simulink model "Project2"  (Simulink 8.0)
settings: Solver=ode23s  StartTime=0.0  StopTime=600  RelTol=1e-4
values from neighbouring files (symbols this model uses):
  a_1 = X(1)    [Init_Project1.m]
  a_2 = X(2)    [Init_Project1.m]
  a_3 = X(3)    [Init_Project1.m]
  A_max_wg = 0.035^2/4*pi    (= 0.000962112750162)    [Init_Project2.m]
  AFS = EngineMap.airfuel.AFs    [Init_Project1.m]
  alpha_REF_manual = 0    [Init_Project2.m]
  alphaEND = alphaINI    (= 0.1)    [Init_Project2.m]
  alphaINI = 0.1    [Init_Project2.m]
  alphaST = 0    [Init_Project2.m]
  BSR_max = turbin_efficiency_parameters(2)    [Init_Project2.m]
  c = sol(1)*(n_cyl/n_r)    [Init_Project1.m]
  C_d = x(3)    [Init_Project1.m]
  C_exh = mean(C_mat)    [Init_Project1.m]
  C_p = A\BMEP    [Init_Project2.m]
  c_p = cp_air    [Init_Project2.m]
  c_r1 = x(1)    [Init_Project1.m]
  c_r2 = x(2)    [Init_Project1.m]
  c_tc_fric = 1e-6    (= 1e-06)    [Init_Project2.m]
  Cd_wg = 0.9    [Init_Project2.m]
  comp_para2 = lsqcurvefit(fn2,[1 1 1 0.8 0.07 1.5], xdata, ydata)    [Init_Project2.m]
  cp_air = gamma_air*cv_air    (= 1213.33333333)    [Init_Project1.m]
  cp_exh = gamma_exh*cv_exh    (= 980)    [Init_Project1.m]
  cyl_sol = A\B    [Init_Project1.m]
  dC2 = 56e-03    (= 0.056)    [Init_Project2.m]
  dP_thrREF = 10e3    (= 10000)    [Init_Project2.m]
  dT1 = 52e-03    (= 0.052)    [Init_Project2.m]
  epsilon = 0.01    [Init_Project2.m]
  eta_T_max = turbin_efficiency_parameters(1)    [Init_Project2.m]
  gamma_air = 1.3    [Init_Project1.m]
  gamma_exh = 1.4    [Init_Project1.m]
  J_tc = 2.55e-5    (= 2.55e-05)    [Init_Project1.m]    (also in Init_Project2.m)
  k_inj = sol(1)    [Init_Project1.m]
  KiDriver = 0.02    [Init_Project1.m]
  KiFuel = 0.02    [Init_Project2.m]
  KpDriver = 0.04    [Init_Project1.m]
  KpFuel = 0.009    [Init_Project2.m]
  KpThr = 1e-6    (= 1e-06)    [Init_Project2.m]
  KpWg = 1e-6    (= 1e-06)    [Init_Project2.m]
  m_dot_c_corr_max = comp_para1(2)    [Init_Project2.m]
  n_cyl = 4    [Init_Project1.m]
  N_e_manual = 0    [Init_Project2.m]
  N_e_step = 1    [Init_Project2.m]
  n_r = 2    [Init_Project1.m]    (also in Init_Project2.m)
  n_vol_parameters = C\D    [Init_Project1.m]
  NEND = NINI    (= 2500)    [Init_Project2.m]
  NeRampInit = 800    [Init_Project2.m]
  NeSlope = 1    [Init_Project2.m]
  NeST = 30    [Init_Project2.m]
  NINI = 2500    [Init_Project2.m]
  p_amb = 101.3e3    (= 101300)    [Init_Project1.m]
  p_ref = comp.pCref    [Init_Project2.m]
  pedEND = 1    [Init_Project2.m]
  pedINI = 0    [Init_Project2.m]
  pedPos_manual = 0    [Init_Project2.m]
  pedST = 30    [Init_Project2.m]
  Psi_max = comp_para1(1)    [Init_Project2.m]
  q_HV = 44e6    (= 44000000)    [Init_Project1.m]
  R_air = 280    [Init_Project1.m]
  r_c = 9.3    [Init_Project1.m]
  R_exh = 280    [Init_Project1.m]
  rho_air = p_amb/(R_air*T_amb)    (= 1.23476352999)    [Init_Project1.m]
  t_0 = sol(2)/sol(1)    [Init_Project1.m]
  T_amb = 293    [Init_Project1.m]
  T_befthr = mean(T_befthr)    [Init_Project1.m]
  T_em = mean(T_em)    [Init_Project1.m]    (also in Init_Project2.m = turb.T03)
  T_ic = mean(T_amb./eta_c(1:34).*(Pi_c.^((gamma_air-1)/gamma_air)-ones(size(Pi_c))+eta_c(1:34)))    [Init_Project2.m]
  T_im = mean(T_im)    [Init_Project1.m]
  T_ref = comp.TCref    [Init_Project2.m]
  T_t = mean(T_em*(1-eta_T.*(1-Pi_T.^((gamma_exh-1)/gamma_exh))))    [Init_Project2.m]
  tau_d = 0.38    [Init_Project1.m]
  tau_mix = 0.1    [Init_Project1.m]
  Tau_th = T*3    [Init_Project1.m]
  tau_wg = 0.07    [Init_Project2.m]
  TFP_exp = turbine_parameters(2)    [Init_Project2.m]
  TFP_max = turbine_parameters(1)    [Init_Project2.m]
  TiThr = 0.1    [Init_Project2.m]
  TiWg = 1    [Init_Project2.m]
  V_D = 2.290 *10^-3    (= 0.00229)    [Init_Project1.m]    (also in Init_Project2.m = n_cyl*V_d)
  V_d = 2*a*pi*B^2/4    (= 0.000572555261117)    [Init_Project1.m]    (also in Init_Project2.m = B^2/4*pi*s)
  V_em = 2e-3    (= 0.002)    [Init_Project1.m]
  V_es = 10e-3    (= 0.01)    [Init_Project1.m]
  V_ic = 10e-3    (= 0.01)    [Init_Project2.m]
  V_im = 2e-3    (= 0.002)    [Init_Project1.m]
  VehicleArea = 2    [Init_Project1.m]
  VehicleMass = 1520    [Init_Project1.m]
  wg_REF_manual = 0    [Init_Project2.m]
  wgEND = wgINI    (= 1)    [Init_Project2.m]
  wgINI = 1    [Init_Project2.m]
  wgST = 30    [Init_Project2.m]
  WheelRadius = 0.3    [Init_Project1.m]
undefined symbols (not defined in the file or in its folder): magnitude, Newton, Raphson, TqEvsNe
libraries: simulink x1
(part 2 of 2)

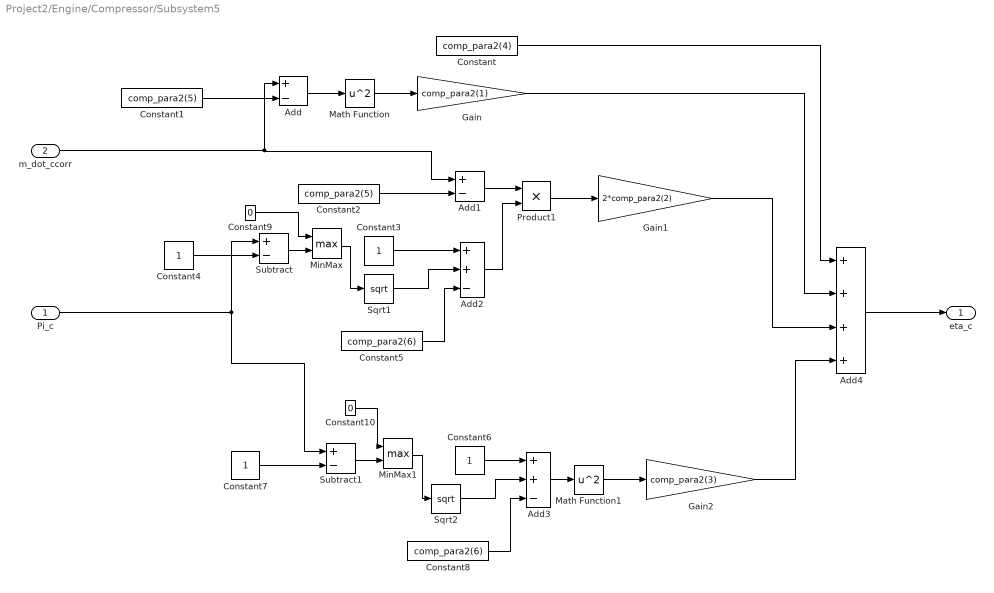
== system Project2/Engine/Compressor/Subsystem5 ==
  Pi_c : Inport
  m_dot_ccorr : Inport  Port=2
  Add : Sum  Inputs=+-
  Add1 : Sum  Inputs=+-
  Add2 : Sum  Inputs=++-
  Add3 : Sum  Inputs=++-
  Add4 : Sum  Inputs=++++
  Constant : Constant  Value=comp_para2(4)
  Constant1 : Constant  Value=comp_para2(5)
  Constant10 : Constant  Value=0
  Constant2 : Constant  Value=comp_para2(5)
  Constant{3..4,6..7} (4 alike) : Constant
  Constant5 : Constant  Value=comp_para2(6)
  Constant8 : Constant  Value=comp_para2(6)
  Constant9 : Constant  Value=0
  Gain : Gain  Gain=comp_para2(1)
  Gain1 : Gain  Gain=2*comp_para2(2)
  Gain2 : Gain  Gain=comp_para2(3)
  Math Function : Math  Operator=square  SaturateOnIntegerOverflow=on
  Math Function1 : Math  Operator=square  SaturateOnIntegerOverflow=on
  MinMax : MinMax  Function=max  Inputs=2
  MinMax1 : MinMax  Function=max  Inputs=2
  Product1 : Product  RndMeth=Zero
  Sqrt1 : Sqrt  SaturateOnIntegerOverflow=on
  Sqrt2 : Sqrt  SaturateOnIntegerOverflow=on
  Subtract : Sum  Inputs=+-
  Subtract1 : Sum  Inputs=+-
  eta_c : Outport
  wires:
  Constant1/1 -> Add/2
  m_dot_ccorr/1 -> Add/1, Add1/1
  Add/1 -> Math Function/1
  Math Function/1 -> Gain/1
  Constant2/1 -> Add1/2
  Add1/1 -> Product1/1
  Product1/1 -> Gain1/1
  Add2/1 -> Product1/2
  Sqrt1/1 -> Add2/2
  Constant3/1 -> Add2/1
  Constant4/1 -> Subtract/2
  Pi_c/1 -> Subtract/1, Subtract1/1
  Constant5/1 -> Add2/3
  Sqrt2/1 -> Add3/2
  Constant6/1 -> Add3/1
  Constant7/1 -> Subtract1/2
  Constant8/1 -> Add3/3
  Add3/1 -> Math Function1/1
  Math Function1/1 -> Gain2/1
  Add4/1 -> eta_c/1
  Gain2/1 -> Add4/4
  Gain1/1 -> Add4/3
  Gain/1 -> Add4/2
  Constant/1 -> Add4/1
  Constant9/1 -> MinMax/1
  Constant10/1 -> MinMax1/1
  Subtract1/1 -> MinMax1/2
  MinMax1/1 -> Sqrt2/1
  Subtract/1 -> MinMax/2
  MinMax/1 -> Sqrt1/1

== system Project2/Engine/Cylinder/Cylinder ==
  m_dot_fc : Inport
  m_dot_ac : Inport  Port=2
  p_em : Inport  Port=3
  p_im : Inport  Port=4
  N : Inport  Port=5
  Add : Sum  Inputs=+--
  Gain : Gain  Gain=1/(2*pi*n_r)
  Subsystem : Subsystem
  Subsystem1 : Subsystem
  w_ig : Subsystem
  M : Outport
  wires:
  m_dot_fc/1 -> w_ig/1(m_dot_fi)
  m_dot_ac/1 -> w_ig/2(m_dot_ac)
  Gain/1 -> M/1
  w_ig/1(W_ig) -> Add/1
  Subsystem/1(w_pump) -> Add/2
  Subsystem1/1(W_fric) -> Add/3
  Add/1 -> Gain/1
  p_im/1 -> Subsystem/2(p_im)
  p_em/1 -> Subsystem/1(p_em)
  N/1 -> w_ig/3(N), Subsystem1/1(N)

== system Project2/Engine/Cylinder/Subsystem1 ==
  m_dot_ac : Inport
  m_dot_fi : Inport  Port=2
  EngineTorque1 : ToWorkspace  VariableName=lambda_cyl  SampleTime=-1
  Gain : Gain  Gain=1/tau_mix
  Integrator : Integrator  InitialCondition=1
  Subsystem : Subsystem
  Subtract : Sum  Inputs=+-
  Transport Delay : TransportDelay  DelayTime=tau_d  InitialOutput=1
  lambda_exh : Outport
  wires:
  Subsystem/1(lambda_cyl) -> EngineTorque1/1, Transport Delay/1
  m_dot_fi/1 -> Subsystem/2(m_dot_fi)
  m_dot_ac/1 -> Subsystem/1(m_dot_ac)
  Transport Delay/1 -> Subtract/1
  Subtract/1 -> Gain/1
  Gain/1 -> Integrator/1
  Integrator/1 -> lambda_exh/1, Subtract/2

== system Project2/Engine/Lambda sensors/Sensor dynamics ==
  lambda : Inport
  Gain1 : Gain  Gain=1/tau_d
  Integrator1 : Integrator  InitialCondition=1
  Subtract1 : Sum  Inputs=+-
  lambda_s : Outport
  wires:
  Gain1/1 -> Integrator1/1
  Subtract1/1 -> Gain1/1
  Integrator1/1 -> Subtract1/2, lambda_s/1
  lambda/1 -> Subtract1/1

== system Project2/Engine/Luftmassflöde till cylinder/Subsystem ==
  N : Inport
  p_im : Inport  Port=2
  Sqrt : Sqrt  SaturateOnIntegerOverflow=on
  Sqrt1 : Sqrt  SaturateOnIntegerOverflow=on
  c0 : Constant  Value=n_vol_parameters(1)
  c1 : Gain  Gain=n_vol_parameters(2)
  c2 : Gain  Gain=n_vol_parameters(3)
  n_vol1 : Sum  Inputs=+++
  n_vol : Outport
  wires:
  Sqrt/1 -> c2/1
  Sqrt1/1 -> c1/1
  c0/1 -> n_vol1/1
  c2/1 -> n_vol1/2
  c1/1 -> n_vol1/3
  N/1 -> Sqrt/1
  n_vol1/1 -> n_vol/1
  p_im/1 -> Sqrt1/1

== system Project2/Engine/Trottel FlÃ¶de/Subsystem1 ==
  alfa_thr : Inport
  p_im : Inport  Port=2
  p_bef_thr : Inport  Port=3
  Constant : Constant  Value=T_befthr
  Gain : Gain  Gain=R_air
  Product2 : Product  Inputs=3  RndMeth=Zero
  Product3 : Product  RndMeth=Zero
  Psi : Subsystem
  Reciprocal Sqrt : Sqrt  Operator=rSqrt  SaturateOnIntegerOverflow=on
  Scope : Scope
      settings: SaveName=ScopeData19
  Scope1 : Scope  NumInputPorts=2
      settings: YMin=-5~-5  YMax=5~5  SaveName=ScopeData17
  Subsystem : Subsystem
  m_dot_at : Outport
  wires:
  p_bef_thr/1 -> Scope1/2, Product3/1, Psi/2(p_bef_thr)
  Psi/1(Psi) -> Scope/1, Product2/2
  Subsystem/1(A_eff) -> Product2/1
  Product3/1 -> Product2/3
  Reciprocal Sqrt/1 -> Product3/2
  Gain/1 -> Reciprocal Sqrt/1
  alfa_thr/1 -> Subsystem/1(alfa_thr)
  Product2/1 -> m_dot_at/1
  p_im/1 -> Scope1/1, Psi/1(p_im)
  Constant/1 -> Gain/1

== system Project2/Engine/Turbine/Subsystem ==
  p04 : Inport
  p03 : Inport  Port=2
  T_em : Inport  Port=3
  "Pa -> kPa" : Gain  Gain=1/1000
  Product : Product  Inputs=3
  Reciprocal Sqrt : Sqrt  Operator=rSqrt  SaturateOnIntegerOverflow=on
  Scope : Scope
      settings: YMin=0.001  YMax=0.0055  SaveName=ScopeData5
  TFP_mod : Subsystem
  mdot_t : Outport
  wires:
  Reciprocal Sqrt/1 -> Product/3
  T_em/1 -> Reciprocal Sqrt/1
  TFP_mod/1(TFP_mod) -> Scope/1, Product/2
  p03/1 -> "Pa -> kPa"/1, TFP_mod/2(p03)
  p04/1 -> TFP_mod/1(p04)
  Product/1 -> mdot_t/1
  "Pa -> kPa"/1 -> Product/1

== system Project2/Engine/Turbine/Subsystem6 ==
  mdot_t : Inport
  T_em : Inport  Port=2
  w_tc : Inport  Port=3
  p_em : Inport  Port=4
  p_t : Inport  Port=5
  N_tc : Inport  Port=6
  Subsystem2 : Subsystem
  Subsystem3 : Subsystem
  Subsystem4 : Subsystem
  Subsystem5 : Subsystem
  Tq_t : Outport
  wires:
  mdot_t/1 -> Subsystem5/2(mdot_t)
  w_tc/1 -> Subsystem5/3(w_tc)
  Subsystem5/1(Tqt) -> Tq_t/1
  Subsystem4/1(T_t) -> Subsystem5/1(T_t)
  Subsystem3/1(eta_t) -> Subsystem4/4(eta_t)
  Subsystem2/1(BSR) -> Subsystem3/1(BSR)
  N_tc/1 -> Subsystem2/4(N_tc)
  p_t/1 -> Subsystem4/2(p_t), Subsystem2/2(p_t)
  p_em/1 -> Subsystem2/1(p_em), Subsystem4/1(p_em)
  T_em/1 -> Subsystem2/3(T_em), Subsystem4/3(T_em), Subsystem5/4(T_em)

== system Project2/Engine/Wastegate/Subsystem1 ==
  alfa_wg : Inport
  p_t : Inport  Port=2
  p_bef_wg : Inport  Port=3
  T_bef_wg : Inport  Port=4
  R_exh : Inport  Port=5
  Aeff_wg : Gain  Gain=Cd_wg*A_max_wg
  Product : Product
  Product2 : Product  Inputs=3  RndMeth=Zero
  Product3 : Product  RndMeth=Zero
  Psi : Subsystem
  Reciprocal Sqrt : Sqrt  Operator=rSqrt  SaturateOnIntegerOverflow=on
  Scope : Scope  NumInputPorts=3
      settings: YMin=-5~-5~-5  YMax=5~5~5  SaveName=ScopeData19
  Scope1 : Scope  NumInputPorts=2
      settings: YMin=-5~-5  YMax=5~5  SaveName=ScopeData17
  m_dot_wg : Outport
  wires:
  p_bef_wg/1 -> Scope1/2, Product3/1, Psi/2(p_bef_wg)
  Psi/1(Psi) -> Scope/2, Product2/2
  Aeff_wg/1 -> Scope/1, Product2/1
  Product3/1 -> Scope/3, Product2/3
  Reciprocal Sqrt/1 -> Product3/2
  Product/1 -> Reciprocal Sqrt/1
  alfa_wg/1 -> Aeff_wg/1
  Product2/1 -> m_dot_wg/1
  p_t/1 -> Scope1/1, Psi/1(p_t)
  T_bef_wg/1 -> Product/1
  R_exh/1 -> Product/2

== system Project2/ECU/Boost Cont/Driver gas pedal interpretation/BMEP -> p_im ==
  BMEP_ref : Inport
  Constant : Constant  Value=C_p(1)
  Gain2 : Gain  Gain=1/C_p(2)
  Subtract2 : Sum
  p_im_ref : Outport
  wires:
  Subtract2/1 -> Gain2/1
  Gain2/1 -> p_im_ref/1
  BMEP_ref/1 -> Subtract2/1
  Constant/1 -> Subtract2/2

== system Project2/ECU/Boost Cont/Throttle Feed Forward/A_eff  ==
  mdot_ac : Inport
  p_imREF : Inport  Port=2
  pbef : Inport  Port=3
  Constant : Constant  Value=epsilon
  Divide : Product  Inputs=*/
  Divide1 : Product  Inputs=*/
  Gain : Gain  Gain=sqrt(R_air*T_ic)
  MinMax : MinMax  Function=max  Inputs=2
  MinMax1 : MinMax  Function=max  Inputs=2
  Product : Product  RndMeth=Zero
  Psi(PI) : Subsystem
  A_eff : Outport
  wires:
  Divide/1 -> Psi(PI)/1(PI)
  MinMax/1 -> Divide/2
  Divide1/1 -> Gain/1
  Product/1 -> Divide1/2
  p_imREF/1 -> Divide/1, MinMax/1
  Gain/1 -> A_eff/1
  pbef/1 -> Product/2, MinMax/2
  Psi(PI)/1(Psi) -> MinMax1/2
  mdot_ac/1 -> Divide1/1
  Constant/1 -> MinMax1/1
  MinMax1/1 -> Product/1

== system Project2/ECU/Boost Cont/Throttle Feed Forward/Aeff ->alpha_thr ==
  A_eff : Inport
  Add : Sum
  Add1 : Sum
  Add2 : Sum  Inputs=+-
  Constant : Constant  Value=0
  Constant1 : Constant  Value=a_1
  Constant2 : Constant  Value=-a_1/(2*a_3)
  Constant3 : Constant  Value=a_2/(2*a_3)
  Gain : Gain  Gain=1/a_3
  Math Function : Math  Operator=square  SaturateOnIntegerOverflow=on
  MinMax : MinMax  Function=max  Inputs=2
  Sqrt : Sqrt  SaturateOnIntegerOverflow=on
  alpha_thr : Outport
  wires:
  Constant1/1 -> Add2/2
  Gain/1 -> Add1/1
  Sqrt/1 -> Add/1
  Constant2/1 -> Add/2
  Math Function/1 -> Add1/2
  A_eff/1 -> Add2/1
  Constant3/1 -> Math Function/1
  Add/1 -> alpha_thr/1
  Add1/1 -> Sqrt/1
  Constant/1 -> MinMax/2
  Add2/1 -> MinMax/1
  MinMax/1 -> Gain/1

== system Project2/ECU/Boost Cont/Throttle Feed Forward/Luftmassflöde till cylinder ==
  N : Inport
  p_im : Inport  Port=2
  Divide : Product  Inputs=*/
  Divide1 : Product  Inputs=***
  Gain : Gain  Gain=(V_d*n_cyl)/(n_r*R_air)
  Subsystem : Subsystem
  T_im : Constant  Value=T_im
  m_dot_ac : Outport
  wires:
  N/1 -> Divide1/3, Subsystem/1(N)
  p_im/1 -> Divide1/2, Subsystem/2(p_im)
  Subsystem/1(n_vol) -> Divide1/1
  Divide1/1 -> Divide/1
  Divide/1 -> Gain/1
  Gain/1 -> m_dot_ac/1
  T_im/1 -> Divide/2

== system Project2/ECU/Fuel Controller/Luftmassflöde till cylinder/Subsystem ==
  N : Inport
  p_im : Inport  Port=2
  Sqrt : Sqrt  SaturateOnIntegerOverflow=on
  Sqrt1 : Sqrt  SaturateOnIntegerOverflow=on
  c0 : Constant  Value=n_vol_parameters(1)*0.96
  c1 : Gain  Gain=n_vol_parameters(2)*1.02
  c2 : Gain  Gain=n_vol_parameters(3)*1.04
  n_vol1 : Sum  Inputs=+++
  n_vol : Outport
  wires:
  Sqrt/1 -> c2/1
  Sqrt1/1 -> c1/1
  c0/1 -> n_vol1/1
  c2/1 -> n_vol1/2
  c1/1 -> n_vol1/3
  N/1 -> Sqrt/1
  n_vol1/1 -> n_vol/1
  p_im/1 -> Sqrt1/1

== system Project2/Engine/Cylinder/Cylinder/Subsystem ==
  p_em : Inport
  p_im : Inport  Port=2
  Gain : Gain  Gain=V_D
  Subtract : Sum  Inputs=+-
  w_pump : Outport
  wires:
  Subtract/1 -> Gain/1
  p_em/1 -> Subtract/1
  Gain/1 -> w_pump/1
  p_im/1 -> Subtract/2

== system Project2/Engine/Cylinder/Cylinder/Subsystem1 ==
  N : Inport
  60/1000 : Gain  Gain=60/1000
  Add : Sum  Inputs=+++
  C_fr,0 : Constant  Value=cyl_sol(2)
  Gain : Gain  Gain=V_D
  Gain1 : Gain  Gain=cyl_sol(4)
  Gain2 : Gain  Gain=cyl_sol(3)
  Math Function : Math  Operator=magnitude^2  SaturateOnIntegerOverflow=on
  W_fric : Outport
  wires:
  60/1000/1 -> Math Function/1, Gain2/1
  Math Function/1 -> Gain1/1
  Gain1/1 -> Add/1
  Gain2/1 -> Add/2
  C_fr,0/1 -> Add/3
  Add/1 -> Gain/1
  N/1 -> 60/1000/1
  Gain/1 -> W_fric/1

== system Project2/Engine/Cylinder/Cylinder/w_ig ==
  m_dot_fi : Inport
  m_dot_ac : Inport  Port=2
  N : Inport  Port=3
  Divide : Product  Inputs=*/
  Gain : Gain  Gain=q_HV*(1-1/r_c^(gamma_air-1))*cyl_sol(1)
  Gain1 : Gain  Gain=n_r
  Lambda : Subsystem
  MinMax : MinMax  Inputs=2
  One : Constant
  W_ : Product  RndMeth=Zero
  W_ig : Outport
  wires:
  m_dot_fi/1 -> Lambda/1(m_fi), Divide/1
  Lambda/1(Lambda) -> MinMax/1
  One/1 -> MinMax/2
  MinMax/1 -> Gain/1
  Gain/1 -> W_/2
  m_dot_ac/1 -> Lambda/2(m_ac)
  W_/1 -> W_ig/1
  N/1 -> Divide/2
  Divide/1 -> Gain1/1
  Gain1/1 -> W_/1

== system Project2/Engine/Cylinder/Subsystem1/Subsystem ==
  m_dot_ac : Inport
  m_dot_fi : Inport  Port=2
  Divide : Product  Inputs=*/
  Gain : Gain  Gain=1/AFS
  lambda_cyl : Outport
  wires:
  Gain/1 -> lambda_cyl/1
  Divide/1 -> Gain/1
  m_dot_fi/1 -> Divide/2
  m_dot_ac/1 -> Divide/1

== system Project2/Engine/Trottel FlÃ¶de/Subsystem1/Psi ==
  p_im : Inport
  p_bef_thr : Inport  Port=2
  Pi : Product  Inputs=*/
  Psi(PI) : Subsystem
  Psi : Outport
  wires:
  Pi/1 -> Psi(PI)/1(PI)
  p_im/1 -> Pi/1
  p_bef_thr/1 -> Pi/2
  Psi(PI)/1(Psi) -> Psi/1

== system Project2/Engine/Trottel FlÃ¶de/Subsystem1/Subsystem ==
  alfa_thr : Inport
  Add : Sum  Inputs=+++
  Product1 : Product  RndMeth=Zero
  a_0 : Gain  Gain=a_1
  a_1 : Gain  Gain=a_2
  a_2 : Gain  Gain=a_3
  one : Constant
  A_eff : Outport
  wires:
  one/1 -> a_0/1
  Product1/1 -> a_2/1
  a_0/1 -> Add/1
  a_1/1 -> Add/2
  a_2/1 -> Add/3
  alfa_thr/1 -> Product1/2, Product1/1, a_1/1
  Add/1 -> A_eff/1

== system Project2/Engine/Turbine/Subsystem/TFP_mod ==
  p04 : Inport
  p03 : Inport  Port=2
  Add : Sum  Inputs=-+
  Constant2 : Constant
  Constant3 : Constant  Value=TFP_exp
  Constant4 : Constant
  Divide : Product  Inputs=*/
  Gain : Gain  Gain=TFP_max
  Math Function : Math  Operator=pow  SaturateOnIntegerOverflow=on
  Pi_t : Product  Inputs=*/
  Scope : Scope
      settings: SaveName=ScopeData7
  Sqrt : Sqrt  SaturateOnIntegerOverflow=on
  TFP_mod : Outport
  wires:
  p03/1 -> Pi_t/1
  p04/1 -> Pi_t/2
  Constant2/1 -> Divide/1
  Divide/1 -> Math Function/1
  Constant3/1 -> Math Function/2
  Constant4/1 -> Add/2
  Gain/1 -> TFP_mod/1
  Sqrt/1 -> Gain/1
  Math Function/1 -> Add/1
  Pi_t/1 -> Divide/2, Scope/1  "PI"
  Add/1 -> Sqrt/1

== system Project2/Engine/Turbine/Subsystem6/Subsystem2 ==
  p_em : Inport
  p_t : Inport  Port=2
  T_em : Inport  Port=3
  N_tc : Inport  Port=4
  Constant : Constant  Value=(gamma_exh-1)/gamma_exh
  Constant1 : Constant
  Divide1 : Product  Inputs=*/
  Divide2 : Product  Inputs=/*
  Gain : Gain  Gain=2*cp_exh
  Gain1 : Gain  Gain=dT1/2
  Math Function : Math  Operator=pow  SaturateOnIntegerOverflow=on
  Pi_t : Product  Inputs=*/
  Product : Product  RndMeth=Zero
  Sqrt : Sqrt  SaturateOnIntegerOverflow=on
  Subtract : Sum  Inputs=+-
  BSR : Outport
  wires:
  Pi_t/1 -> Math Function/1
  Constant/1 -> Math Function/2
  Math Function/1 -> Divide1/2
  Constant1/1 -> Subtract/1, Divide1/1
  Divide1/1 -> Subtract/2
  Product/1 -> Sqrt/1
  Subtract/1 -> Product/2
  Gain/1 -> Product/1
  T_em/1 -> Gain/1
  Sqrt/1 -> Divide2/1
  Divide2/1 -> BSR/1
  Gain1/1 -> Divide2/2
  N_tc/1 -> Gain1/1
  p_t/1 -> Pi_t/2
  p_em/1 -> Pi_t/1

== system Project2/Engine/Turbine/Subsystem6/Subsystem3 ==
  BSR : Inport
  Constant : Constant
  Constant1 : Constant  Value=BSR_max
  Gain : Gain  Gain=eta_T_max
  Gain1 : Gain  Gain=1/BSR_max
  Math Function : Math  Operator=square  SaturateOnIntegerOverflow=on
  MinMax : MinMax  Inputs=2
  Subtract : Sum  Inputs=+-
  Subtract1 : Sum  Inputs=+-
  eta_t : Outport
  wires:
  Gain/1 -> eta_t/1
  Subtract/1 -> Gain/1
  Constant/1 -> Subtract/1
  Math Function/1 -> Subtract/2
  Gain1/1 -> Math Function/1
  Subtract1/1 -> Gain1/1
  Constant1/1 -> MinMax/2, Subtract1/2
  BSR/1 -> MinMax/1
  MinMax/1 -> Subtract1/1

== system Project2/Engine/Turbine/Subsystem6/Subsystem4 ==
  p_em : Inport
  p_t : Inport  Port=2
  T_em : Inport  Port=3
  eta_t : Inport  Port=4
  Constant : Constant  Value=(gamma_exh-1)/gamma_exh
  Constant1 : Constant
  Constant2 : Constant
  Math Function : Math  Operator=pow  SaturateOnIntegerOverflow=on
  Pi_t : Product  Inputs=*/
  Product : Product  RndMeth=Zero
  Product1 : Product  RndMeth=Zero
  Subtract : Sum  Inputs=+-
  Subtract1 : Sum  Inputs=+-
  T_t : Outport
  wires:
  p_t/1 -> Pi_t/1
  p_em/1 -> Pi_t/2
  Pi_t/1 -> Math Function/1
  Constant/1 -> Math Function/2
  Constant1/1 -> Subtract/1
  Math Function/1 -> Subtract/2
  Subtract/1 -> Product/1
  eta_t/1 -> Product/2
  Constant2/1 -> Subtract1/1
  Product/1 -> Subtract1/2
  Product1/1 -> T_t/1
  Subtract1/1 -> Product1/1
  T_em/1 -> Product1/2

== system Project2/Engine/Turbine/Subsystem6/Subsystem5 ==
  T_t : Inport
  mdot_t : Inport  Port=2
  w_tc : Inport  Port=3
  T_em : Inport  Port=4
  Gain : Gain  Gain=cp_exh
  Product : Product  Inputs=**/  RndMeth=Zero
  Subtract : Sum  Inputs=+-
  Tqt : Outport
  wires:
  w_tc/1 -> Product/3
  mdot_t/1 -> Product/2
  T_t/1 -> Subtract/2
  T_em/1 -> Subtract/1
  Subtract/1 -> Product/1
  Product/1 -> Gain/1
  Gain/1 -> Tqt/1

== system Project2/Engine/Wastegate/Subsystem1/Psi ==
  p_t : Inport
  p_bef_wg : Inport  Port=2
  Pi : Product  Inputs=*/
  Psi(PI) : Subsystem
  Psi : Outport
  wires:
  Pi/1 -> Psi(PI)/1(PI)
  Psi(PI)/1(Psi) -> Psi/1
  p_t/1 -> Pi/1
  p_bef_wg/1 -> Pi/2

== system Project2/ECU/Boost Cont/Throttle Feed Forward/A_eff /Psi(PI) ==
  PI : Inport
  (g+1)/g : Constant  Value=(gamma_air+1)/gamma_air
  2/g : Constant  Value=2/gamma_air
  2g/(g-1) : Constant  Value=(2*gamma_air)/(gamma_air-1)
  Math Function : Math  Operator=pow  SaturateOnIntegerOverflow=on
  Math Function1 : Math  Operator=pow  SaturateOnIntegerOverflow=on
  MinMax : MinMax  Function=max  Inputs=2
  PI critical (2/(g+1))^(g/(g-1)) : Constant  Value=(2/(gamma_air+1))^(gamma_air/(gamma_air-1))
  Product : Product  RndMeth=Zero
  Sqrt : Sqrt  AlgorithmType=Newton-Raphson  SaturateOnIntegerOverflow=on
  Subtract : Sum  Inputs=+-
  "[0,1]" : Saturate  UpperLimit=1  LowerLimit=0
  Psi : Outport
  wires:
  PI/1 -> "[0,1]"/1  "PI"
  PI critical (2/(g+1))^(g/(g-1))/1 -> MinMax/2
  MinMax/1 -> Math Function/1, Math Function1/1  "PIlim"
  2/g/1 -> Math Function/2
  (g+1)/g/1 -> Math Function1/2
  "[0,1]"/1 -> MinMax/1
  Math Function/1 -> Subtract/1
  Math Function1/1 -> Subtract/2
  Subtract/1 -> Product/1
  2g/(g-1)/1 -> Product/2
  Product/1 -> Sqrt/1
  Sqrt/1 -> Psi/1  "Psi"

== system Project2/ECU/Boost Cont/Throttle Feed Forward/Luftmassflöde till cylinder/Subsystem ==
  N : Inport
  p_im : Inport  Port=2
  Sqrt : Sqrt  SaturateOnIntegerOverflow=on
  Sqrt1 : Sqrt  SaturateOnIntegerOverflow=on
  c0 : Constant  Value=n_vol_parameters(1)
  c1 : Gain  Gain=n_vol_parameters(2)
  c2 : Gain  Gain=n_vol_parameters(3)
  n_vol1 : Sum  Inputs=+++
  n_vol : Outport
  wires:
  Sqrt/1 -> c2/1
  Sqrt1/1 -> c1/1
  c0/1 -> n_vol1/1
  c2/1 -> n_vol1/2
  c1/1 -> n_vol1/3
  N/1 -> Sqrt/1
  n_vol1/1 -> n_vol/1
  p_im/1 -> Sqrt1/1

== system Project2/Engine/Cylinder/Cylinder/w_ig/Lambda ==
  m_fi : Inport
  m_ac : Inport  Port=2
  (A/F)_s : Gain  Gain=AFS
  Divide : Product  Inputs=*/
  Lambda : Outport
  wires:
  (A/F)_s/1 -> Divide/2
  m_fi/1 -> (A/F)_s/1
  m_ac/1 -> Divide/1
  Divide/1 -> Lambda/1

== system Project2/Engine/Trottel FlÃ¶de/Subsystem1/Psi/Psi(PI) ==
  PI : Inport
  (g+1)/g : Constant  Value=(gamma_air+1)/gamma_air
  2/g : Constant  Value=2/gamma_air
  2g/(g-1) : Constant  Value=(2*gamma_air)/(gamma_air-1)
  Math Function : Math  Operator=pow  SaturateOnIntegerOverflow=on
  Math Function1 : Math  Operator=pow  SaturateOnIntegerOverflow=on
  MinMax : MinMax  Function=max  Inputs=2
  PI critical (2/(g+1))^(g/(g-1)) : Constant  Value=(2/(gamma_air+1))^(gamma_air/(gamma_air-1))
  Product : Product  RndMeth=Zero
  Sqrt : Sqrt  AlgorithmType=Newton-Raphson  SaturateOnIntegerOverflow=on
  Subtract : Sum  Inputs=+-
  "[0,1]" : Saturate  UpperLimit=1  LowerLimit=0
  Psi : Outport
  wires:
  PI/1 -> "[0,1]"/1  "PI"
  PI critical (2/(g+1))^(g/(g-1))/1 -> MinMax/2
  MinMax/1 -> Math Function/1, Math Function1/1  "PIlim"
  2/g/1 -> Math Function/2
  (g+1)/g/1 -> Math Function1/2
  "[0,1]"/1 -> MinMax/1
  Math Function/1 -> Subtract/1
  Math Function1/1 -> Subtract/2
  Subtract/1 -> Product/1
  2g/(g-1)/1 -> Product/2
  Product/1 -> Sqrt/1
  Sqrt/1 -> Psi/1  "Psi"

== system Project2/Engine/Wastegate/Subsystem1/Psi/Psi(PI) ==
  PI : Inport
  (g+1)/g : Constant  Value=(gamma_exh+1)/gamma_exh
  2/g : Constant  Value=2/gamma_exh
  2g/(g-1) : Constant  Value=(2*gamma_exh)/(gamma_exh-1)
  Math Function : Math  Operator=pow  SaturateOnIntegerOverflow=on
  Math Function1 : Math  Operator=pow  SaturateOnIntegerOverflow=on
  MinMax : MinMax  Function=max  Inputs=2
  PI critical (2/(g+1))^(g/(g-1)) : Constant  Value=(2/(gamma_exh+1))^(gamma_exh/(gamma_exh-1))
  Product : Product  RndMeth=Zero
  Sqrt : Sqrt  AlgorithmType=Newton-Raphson  SaturateOnIntegerOverflow=on
  Subtract : Sum  Inputs=+-
  "[0,1]" : Saturate  UpperLimit=1  LowerLimit=0
  Psi : Outport
  wires:
  PI/1 -> "[0,1]"/1  "PI"
  PI critical (2/(g+1))^(g/(g-1))/1 -> MinMax/2
  MinMax/1 -> Math Function/1, Math Function1/1  "PIlim"
  2/g/1 -> Math Function/2
  (g+1)/g/1 -> Math Function1/2
  "[0,1]"/1 -> MinMax/1
  Math Function/1 -> Subtract/1
  Math Function1/1 -> Subtract/2
  Subtract/1 -> Product/1
  2g/(g-1)/1 -> Product/2
  Product/1 -> Sqrt/1
  Sqrt/1 -> Psi/1  "Psi"
